simulink library "fdclib10"  (Simulink 3.00)
undefined symbols (not defined in the file): GM1
libraries: fdclib6 x3, fdclib4 x2, fdclib10 x2, fdclib2 x1, fdclib5 x1, fdclib1 x1, fdclib3 x1
settings Model: LastModifiedBy=Dutchroll

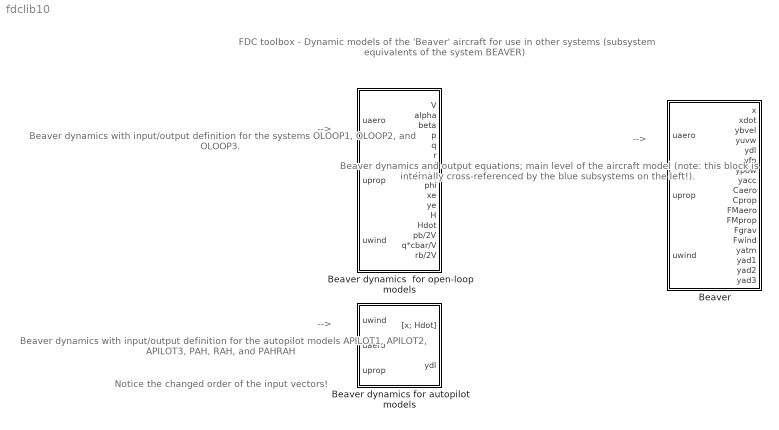
== system fdclib10 ==
  note: -->
  note: -->
  note: Beaver dynamics with input/output
      | definition for the autopilot models
      | APILOT1, APILOT2,  APILOT3,
      | PAH, RAH, and PAHRAH
  note: Beaver dynamics with input/output
      | definition for the systems OLOOP1,
      | OLOOP2, and OLOOP3.
  note: FDC toolbox - Dynamic models of the 'Beaver' aircraft for use in other systems
      | (subsystem equivalents of the system BEAVER)
  note: Beaver dynamics and output
      | equations; main level of the
      | aircraft model (note: this block
      | is internally cross-referenced
      | by the blue subsystems on
      | the left!).
  note: -->
  note: Notice the changed order of
      | the input vectors!
  Beaver : Subsystem
      mask Type: Beaver dynamics and output equations
      mask Description: Nonlinear dynamic model of the De Havilland DHC-2 'Beaver' aircraft, plus additional airdata and flight-path equations.
      mask Help: eval('browse level2')
      mask Display: disp('DeHavilland\nDHC-2 Beaver\ndynamics and\noutput equations');
  Beaver dynamics  for open-loop models : Subsystem
  Beaver dynamics for autopilot models : Subsystem

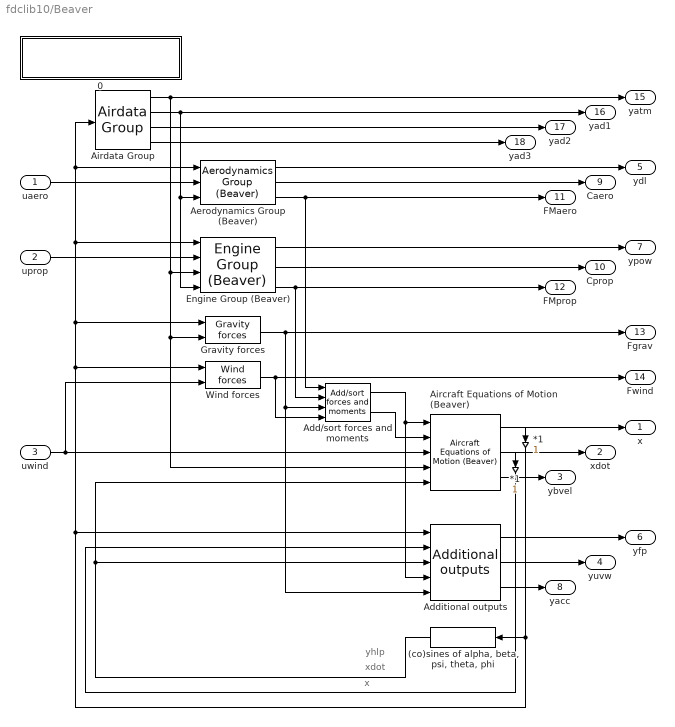
== system fdclib10/Beaver ==
  note: xdot
  note: x
  note: yhlp
  uaero : Inport  Port=1  PortWidth=-1  SampleTime=-1  DataType=auto
      settings: SignalType=auto
  uprop : Inport  Port=2  PortWidth=-1  SampleTime=-1  DataType=auto
      settings: SignalType=auto
  uwind : Inport  Port=3  PortWidth=-1  SampleTime=-1  DataType=auto
      settings: SignalType=auto
  " *1" : Gain  Orientation=down  Gain=1  SaturateOnIntegerOverflow=on
  "(co)sines of alpha, beta, psi, theta, phi" : fdclib6/(co)sines of alpha, beta, psi, theta, phi  Orientation=left
  *1 : Gain  Orientation=down  Gain=1  SaturateOnIntegerOverflow=on
  0 : Subsystem
      settings: OpenFcn=browse level2
      mask Display: disp('BEAVER, level 2 (main level)\nM.O. Rauw, November 2004')
  Add/sort forces and moments : fdclib6/Add//sort forces and moments
  Additional outputs : fdclib6/Additional outputs
  Aerodynamics Group (Beaver) : fdclib2/Aerodynamics Group (Beaver)
  Aircraft Equations of Motion (Beaver) : fdclib5/Aircraft Equations of Motion (Beaver)
  Airdata Group : fdclib1/Airdata Group
  Engine Group (Beaver) : fdclib3/Engine Group (Beaver)
  Gravity forces : fdclib4/Gravity forces  m=GM1(10)
  Wind forces : fdclib4/Wind forces  m=GM1(10)
  x : Outport  Port=1
  xdot : Outport  Port=2
  ybvel : Outport  Port=3
  yuvw : Outport  Port=4
  ydl : Outport  Port=5
  yfp : Outport  Port=6
  ypow : Outport  Port=7
  yacc : Outport  Port=8
  Caero : Outport  Port=9
  Cprop : Outport  Port=10
  FMaero : Outport  Port=11
  FMprop : Outport  Port=12
  Fgrav : Outport  Port=13
  Fwind : Outport  Port=14
  yatm : Outport  Port=15
  yad1 : Outport  Port=16
  yad2 : Outport  Port=17
  yad3 : Outport  Port=18
  wires:
  uprop/1 -> Engine Group (Beaver)/2
  uaero/1 -> Aerodynamics Group (Beaver)/2
  Wind forces/1 -> Fwind/1, Add/sort forces and moments/4
  Engine Group (Beaver)/3 -> FMprop/1, Add/sort forces and moments/2
  Aerodynamics Group (Beaver)/3 -> FMaero/1, Add/sort forces and moments/1
  Gravity forces/1 -> Fgrav/1, Add/sort forces and moments/3, Additional outputs/5
  Add/sort forces and moments/1 -> Additional outputs/4, Aircraft Equations of Motion (Beaver)/1
  Engine Group (Beaver)/2 -> Cprop/1
  Engine Group (Beaver)/1 -> ypow/1
  Aerodynamics Group (Beaver)/1 -> ydl/1
  Aerodynamics Group (Beaver)/2 -> Caero/1
  Airdata Group/2 -> Engine Group (Beaver)/4, Aerodynamics Group (Beaver)/3, yad1/1
  Airdata Group/1 -> yatm/1, Engine Group (Beaver)/3, Aircraft Equations of Motion (Beaver)/4, Gravity forces/2
  Airdata Group/4 -> yad3/1
  Airdata Group/3 -> yad2/1
  uwind/1 -> Aircraft Equations of Motion (Beaver)/3, Wind forces/2
  Add/sort forces and moments/2 -> Aircraft Equations of Motion (Beaver)/2
  Aircraft Equations of Motion (Beaver)/3 -> ybvel/1
  Aircraft Equations of Motion (Beaver)/2 -> xdot/1, *1/1
  Aircraft Equations of Motion (Beaver)/1 -> x/1, " *1"/1
  "(co)sines of alpha, beta, psi, theta, phi"/1 -> Aircraft Equations of Motion (Beaver)/5, Additional outputs/3
  Additional outputs/2 -> yuvw/1
  Additional outputs/1 -> yfp/1
  Additional outputs/3 -> yacc/1
  *1/1 -> Additional outputs/2
  " *1"/1 -> "(co)sines of alpha, beta, psi, theta, phi"/1, Additional outputs/1, Wind forces/1, Gravity forces/1, Engine Group (Beaver)/1, Aerodynamics Group (Beaver)/1, Airdata Group/1

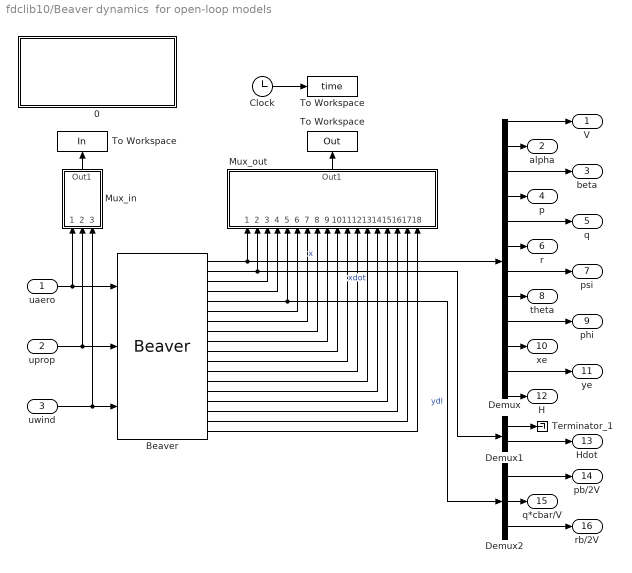
== system fdclib10/Beaver dynamics  for open-loop models ==
  uaero : Inport  Port=1  PortWidth=-1  SampleTime=-1  DataType=auto
      settings: SignalType=auto
  uprop : Inport  Port=2  PortWidth=-1  SampleTime=-1  DataType=auto
      settings: SignalType=auto
  uwind : Inport  Port=3  PortWidth=-1  SampleTime=-1  DataType=auto
      settings: SignalType=auto
  0 : Subsystem
      settings: OpenFcn=browse level1
      mask Display: disp('Beaver dynamics with\nI/O definitions for the\nopen-loop simulation models\nM.O. Rauw, September 2004')
  Beaver : fdclib10/Beaver
  Clock : Clock
      settings: DisplayTime=off  Decimation=10
  Demux : Demux  Outputs=12
  Demux1 : Demux  Outputs=[11 1]
  Demux2 : Demux  Outputs=3
  Mux_in : Subsystem  Orientation=up
      settings: OpenFcn=browse inputs
      mask Display: disp('Mux\nclick\n2x for\ninfo!')
  Mux_out : Subsystem  Orientation=up
      settings: OpenFcn=browse outputs
      mask Display: disp('Mux\n\nDouble-click for info!')
  Terminator_1 : Terminator
  To Workspace : ToWorkspace  VariableName=Out  SampleTime=0  SaveFormat=Matrix
      settings: Orientation=up  Buffer=5000
  "To Workspace " : ToWorkspace  VariableName=In  SampleTime=0  SaveFormat=Matrix
      settings: Orientation=up  Buffer=5000
  "To Workspace  " : ToWorkspace  VariableName=time  SampleTime=0  SaveFormat=Matrix
      settings: Buffer=5000
  V : Outport  Port=1
  alpha : Outport  Port=2
  beta : Outport  Port=3
  p : Outport  Port=4
  q : Outport  Port=5
  r : Outport  Port=6
  psi : Outport  Port=7
  theta : Outport  Port=8
  phi : Outport  Port=9
  xe : Outport  Port=10
  ye : Outport  Port=11
  H : Outport  Port=12
  Hdot : Outport  Port=13
  pb/2V : Outport  Port=14
  q*cbar/V : Outport  Port=15
  rb/2V : Outport  Port=16
  wires:
  uaero/1 -> Mux_in/1(In1), Beaver/1
  uprop/1 -> Mux_in/2(In2), Beaver/2
  uwind/1 -> Mux_in/3(In3), Beaver/3
  Mux_in/1(Out1) -> "To Workspace "/1
  Demux/10 -> xe/1
  Demux/11 -> ye/1
  Demux/12 -> H/1
  Demux/9 -> phi/1
  Demux/8 -> theta/1
  Demux/7 -> psi/1
  Demux/6 -> r/1
  Demux/5 -> q/1
  Demux/4 -> p/1
  Demux/3 -> beta/1
  Demux/2 -> alpha/1
  Demux/1 -> V/1
  Beaver/1 -> Mux_out/1(In1), Demux/1  "x"
  Beaver/18 -> Mux_out/18(In18)
  Beaver/17 -> Mux_out/17(In17)
  Beaver/4 -> Mux_out/4(In4)
  Beaver/3 -> Mux_out/3(In3)
  Beaver/16 -> Mux_out/16(In16)
  Beaver/5 -> Mux_out/5(In5), Demux2/1  "ydl"
  Beaver/6 -> Mux_out/6(In6)
  Beaver/8 -> Mux_out/8(In8)
  Beaver/9 -> Mux_out/9(In9)
  Beaver/10 -> Mux_out/10(In10)
  Beaver/11 -> Mux_out/11(In11)
  Beaver/12 -> Mux_out/12(In12)
  Beaver/13 -> Mux_out/13(In13)
  Beaver/14 -> Mux_out/14(In14)
  Beaver/15 -> Mux_out/15(In15)
  Mux_out/1(Out1) -> To Workspace/1
  Beaver/7 -> Mux_out/7(In7)
  Beaver/2 -> Demux1/1, Mux_out/2(In2)  "xdot"
  Demux1/2 -> Hdot/1
  Demux1/1 -> Terminator_1/1
  Demux2/2 -> q*cbar/V/1
  Demux2/1 -> pb/2V/1
  Demux2/3 -> rb/2V/1
  Clock/1 -> "To Workspace  "/1

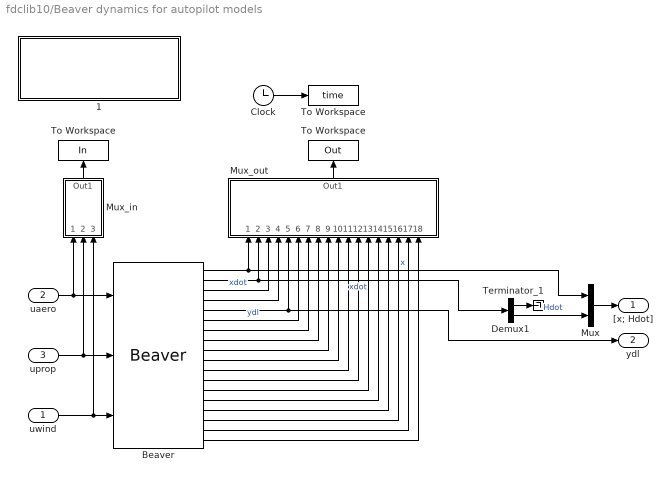
== system fdclib10/Beaver dynamics for autopilot models ==
  uwind : Inport  Port=1  PortWidth=-1  SampleTime=-1  DataType=auto
      settings: SignalType=auto
  uaero : Inport  Port=2  PortWidth=-1  SampleTime=-1  DataType=auto
      settings: SignalType=auto
  uprop : Inport  Port=3  PortWidth=-1  SampleTime=-1  DataType=auto
      settings: SignalType=auto
  1 : Subsystem
      settings: OpenFcn=browse level1
      mask Display: disp('Beaver dynamics with\nI/O definitions for the\nautopilot simulation models\nM.O. Rauw, September 2004')
  Beaver : fdclib10/Beaver
  Clock : Clock
      settings: DisplayTime=off  Decimation=10
  Demux1 : Demux  Outputs=[11 1]
  Mux : Mux  Inputs=[12 1]
      settings: DisplayOption=none
  Mux_in : Subsystem  Orientation=up
      settings: OpenFcn=browse inputs
      mask Display: disp('Mux\nclick\n2x for\ninfo!')
  Mux_out : Subsystem  Orientation=up
      settings: OpenFcn=browse outputs
      mask Display: disp('Mux\n\nDouble-click for info!')
  Terminator_1 : Terminator
  To Workspace : ToWorkspace  VariableName=Out  SampleTime=0  SaveFormat=Matrix
      settings: Orientation=up  Buffer=5000
  "To Workspace " : ToWorkspace  VariableName=In  SampleTime=0  SaveFormat=Matrix
      settings: Orientation=up  Buffer=5000
  "To Workspace  " : ToWorkspace  VariableName=time  SampleTime=0  SaveFormat=Matrix
      settings: Buffer=5000
  "[x; Hdot]" : Outport  Port=1
  ydl : Outport  Port=2
  wires:
  uaero/1 -> Mux_in/1(In1), Beaver/1
  uprop/1 -> Mux_in/2(In2), Beaver/2
  uwind/1 -> Mux_in/3(In3), Beaver/3
  Mux_in/1(Out1) -> "To Workspace "/1
  Beaver/1 -> Mux_out/1(In1), Mux/1  "x"
  Beaver/18 -> Mux_out/18(In18)
  Beaver/17 -> Mux_out/17(In17)
  Beaver/4 -> Mux_out/4(In4)
  Beaver/16 -> Mux_out/16(In16)
  Beaver/8 -> Mux_out/8(In8)
  Beaver/9 -> Mux_out/9(In9)
  Beaver/10 -> Mux_out/10(In10)
  Beaver/11 -> Mux_out/11(In11)
  Beaver/12 -> Mux_out/12(In12)
  Beaver/13 -> Mux_out/13(In13)
  Beaver/14 -> Mux_out/14(In14)
  Beaver/15 -> Mux_out/15(In15)
  Mux_out/1(Out1) -> To Workspace/1
  Beaver/7 -> Mux_out/7(In7)
  Clock/1 -> "To Workspace  "/1
  Mux/1 -> "[x; Hdot]"/1
  Beaver/3 -> Mux_out/3(In3)  "xdot"
  Beaver/2 -> Mux_out/2(In2), Demux1/1  "xdot"
  Beaver/6 -> Mux_out/6(In6)  "ydl"
  Beaver/5 -> Mux_out/5(In5), ydl/1
  Demux1/1 -> Terminator_1/1
  Demux1/2 -> Mux/2  "Hdot"

== system fdclib10/Beaver/0 ==

== system fdclib10/Beaver dynamics  for open-loop models/0 ==

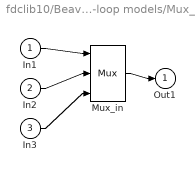
== system fdclib10/Beaver dynamics  for open-loop models/Mux_in ==
  In1 : Inport  Port=1  PortWidth=-1  SampleTime=-1  DataType=auto
      settings: SignalType=auto
  In2 : Inport  Port=2  PortWidth=-1  SampleTime=-1  DataType=auto
      settings: SignalType=auto
  In3 : Inport  Port=3  PortWidth=-1  SampleTime=-1  DataType=auto
      settings: SignalType=auto
  Mux_in : Mux  Inputs=[4 2 6]
      settings: DisplayOption=none
  Out1 : Outport  Port=1
  wires:
  In1/1 -> Mux_in/1
  In2/1 -> Mux_in/2
  In3/1 -> Mux_in/3
  Mux_in/1 -> Out1/1

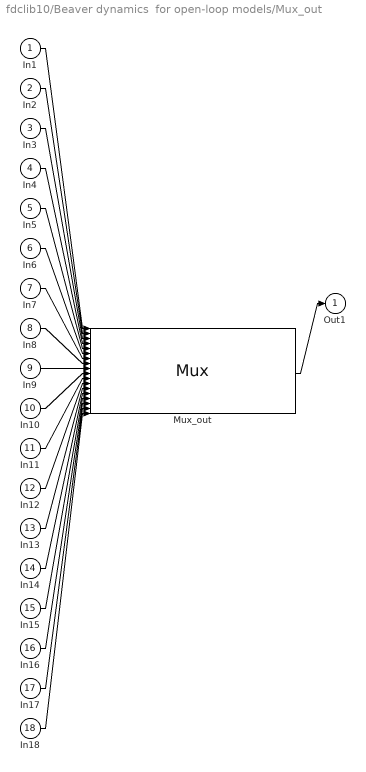
== system fdclib10/Beaver dynamics  for open-loop models/Mux_out ==
  In1 : Inport  Port=1  PortWidth=-1  SampleTime=-1  DataType=auto
      settings: SignalType=auto
  In2 : Inport  Port=2  PortWidth=-1  SampleTime=-1  DataType=auto
      settings: SignalType=auto
  In3 : Inport  Port=3  PortWidth=-1  SampleTime=-1  DataType=auto
      settings: SignalType=auto
  In4 : Inport  Port=4  PortWidth=-1  SampleTime=-1  DataType=auto
      settings: SignalType=auto
  In5 : Inport  Port=5  PortWidth=-1  SampleTime=-1  DataType=auto
      settings: SignalType=auto
  In6 : Inport  Port=6  PortWidth=-1  SampleTime=-1  DataType=auto
      settings: SignalType=auto
  In7 : Inport  Port=7  PortWidth=-1  SampleTime=-1  DataType=auto
      settings: SignalType=auto
  In8 : Inport  Port=8  PortWidth=-1  SampleTime=-1  DataType=auto
      settings: SignalType=auto
  In9 : Inport  Port=9  PortWidth=-1  SampleTime=-1  DataType=auto
      settings: SignalType=auto
  In10 : Inport  Port=10  PortWidth=-1  SampleTime=-1  DataType=auto
      settings: SignalType=auto
  In11 : Inport  Port=11  PortWidth=-1  SampleTime=-1  DataType=auto
      settings: SignalType=auto
  In12 : Inport  Port=12  PortWidth=-1  SampleTime=-1  DataType=auto
      settings: SignalType=auto
  In13 : Inport  Port=13  PortWidth=-1  SampleTime=-1  DataType=auto
      settings: SignalType=auto
  In14 : Inport  Port=14  PortWidth=-1  SampleTime=-1  DataType=auto
      settings: SignalType=auto
  In15 : Inport  Port=15  PortWidth=-1  SampleTime=-1  DataType=auto
      settings: SignalType=auto
  In16 : Inport  Port=16  PortWidth=-1  SampleTime=-1  DataType=auto
      settings: SignalType=auto
  In17 : Inport  Port=17  PortWidth=-1  SampleTime=-1  DataType=auto
      settings: SignalType=auto
  In18 : Inport  Port=18  PortWidth=-1  SampleTime=-1  DataType=auto
      settings: SignalType=auto
  Mux_out : Mux  Inputs=[12 12 3 3 3 4 2 6 6 6 6 6 3 3 5 3 3 3]
      settings: DisplayOption=none
  Out1 : Outport  Port=1
  wires:
  In1/1 -> Mux_out/1
  In2/1 -> Mux_out/2
  In3/1 -> Mux_out/3
  In4/1 -> Mux_out/4
  In5/1 -> Mux_out/5
  In6/1 -> Mux_out/6
  In7/1 -> Mux_out/7
  In8/1 -> Mux_out/8
  In9/1 -> Mux_out/9
  In10/1 -> Mux_out/10
  In11/1 -> Mux_out/11
  In12/1 -> Mux_out/12
  In13/1 -> Mux_out/13
  In14/1 -> Mux_out/14
  In15/1 -> Mux_out/15
  In16/1 -> Mux_out/16
  In17/1 -> Mux_out/17
  In18/1 -> Mux_out/18
  Mux_out/1 -> Out1/1

== system fdclib10/Beaver dynamics for autopilot models/1 ==

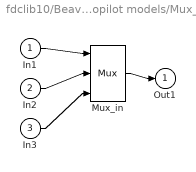
== system fdclib10/Beaver dynamics for autopilot models/Mux_in ==
  In1 : Inport  Port=1  PortWidth=-1  SampleTime=-1  DataType=auto
      settings: SignalType=auto
  In2 : Inport  Port=2  PortWidth=-1  SampleTime=-1  DataType=auto
      settings: SignalType=auto
  In3 : Inport  Port=3  PortWidth=-1  SampleTime=-1  DataType=auto
      settings: SignalType=auto
  Mux_in : Mux  Inputs=[4 2 6]
      settings: DisplayOption=none
  Out1 : Outport  Port=1
  wires:
  Mux_in/1 -> Out1/1
  In3/1 -> Mux_in/3
  In2/1 -> Mux_in/2
  In1/1 -> Mux_in/1

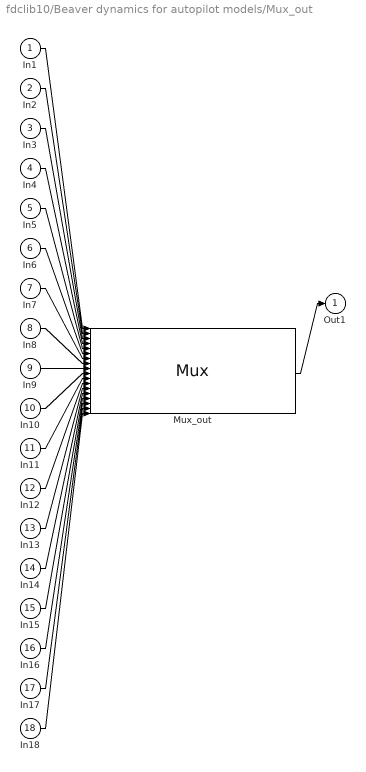
== system fdclib10/Beaver dynamics for autopilot models/Mux_out ==
  In1 : Inport  Port=1  PortWidth=-1  SampleTime=-1  DataType=auto
      settings: SignalType=auto
  In2 : Inport  Port=2  PortWidth=-1  SampleTime=-1  DataType=auto
      settings: SignalType=auto
  In3 : Inport  Port=3  PortWidth=-1  SampleTime=-1  DataType=auto
      settings: SignalType=auto
  In4 : Inport  Port=4  PortWidth=-1  SampleTime=-1  DataType=auto
      settings: SignalType=auto
  In5 : Inport  Port=5  PortWidth=-1  SampleTime=-1  DataType=auto
      settings: SignalType=auto
  In6 : Inport  Port=6  PortWidth=-1  SampleTime=-1  DataType=auto
      settings: SignalType=auto
  In7 : Inport  Port=7  PortWidth=-1  SampleTime=-1  DataType=auto
      settings: SignalType=auto
  In8 : Inport  Port=8  PortWidth=-1  SampleTime=-1  DataType=auto
      settings: SignalType=auto
  In9 : Inport  Port=9  PortWidth=-1  SampleTime=-1  DataType=auto
      settings: SignalType=auto
  In10 : Inport  Port=10  PortWidth=-1  SampleTime=-1  DataType=auto
      settings: SignalType=auto
  In11 : Inport  Port=11  PortWidth=-1  SampleTime=-1  DataType=auto
      settings: SignalType=auto
  In12 : Inport  Port=12  PortWidth=-1  SampleTime=-1  DataType=auto
      settings: SignalType=auto
  In13 : Inport  Port=13  PortWidth=-1  SampleTime=-1  DataType=auto
      settings: SignalType=auto
  In14 : Inport  Port=14  PortWidth=-1  SampleTime=-1  DataType=auto
      settings: SignalType=auto
  In15 : Inport  Port=15  PortWidth=-1  SampleTime=-1  DataType=auto
      settings: SignalType=auto
  In16 : Inport  Port=16  PortWidth=-1  SampleTime=-1  DataType=auto
      settings: SignalType=auto
  In17 : Inport  Port=17  PortWidth=-1  SampleTime=-1  DataType=auto
      settings: SignalType=auto
  In18 : Inport  Port=18  PortWidth=-1  SampleTime=-1  DataType=auto
      settings: SignalType=auto
  Mux_out : Mux  Inputs=[12 12 3 3 3 4 2 6 6 6 6 6 3 3 5 3 3 3]
      settings: DisplayOption=none
  Out1 : Outport  Port=1
  wires:
  Mux_out/1 -> Out1/1
  In18/1 -> Mux_out/18
  In17/1 -> Mux_out/17
  In16/1 -> Mux_out/16
  In15/1 -> Mux_out/15
  In14/1 -> Mux_out/14
  In13/1 -> Mux_out/13
  In12/1 -> Mux_out/12
  In11/1 -> Mux_out/11
  In10/1 -> Mux_out/10
  In9/1 -> Mux_out/9
  In8/1 -> Mux_out/8
  In7/1 -> Mux_out/7
  In6/1 -> Mux_out/6
  In5/1 -> Mux_out/5
  In4/1 -> Mux_out/4
  In3/1 -> Mux_out/3
  In2/1 -> Mux_out/2
  In1/1 -> Mux_out/1
